simulink model "Inversor_full_bridge_ma"  (R2015a)
settings: Solver=ode23tb  StartTime=0.0  StopTime=0.2  MaxStep=0.5e-6  RelTol=1e-3
libraries: powerlib x11, simulink x1
settings Model: Creator=Leandro  LastModifiedBy=Iury
settings DataIOCC: SignalLoggingSaveFormat=ModelDataLogs
settings DebuggingCC: UnderspecifiedInitializationDetection=Classic  MergeDetectMultiDrivingBlocksExec=none  SolverPrmCheckMsg=warning  FcnCallInpInsideContextMsg=UseLocalSettings  StateNameClashWarn=warning
settings GRTTargetCC: CombineOutputUpdateFcns=off  GRTInterface=on

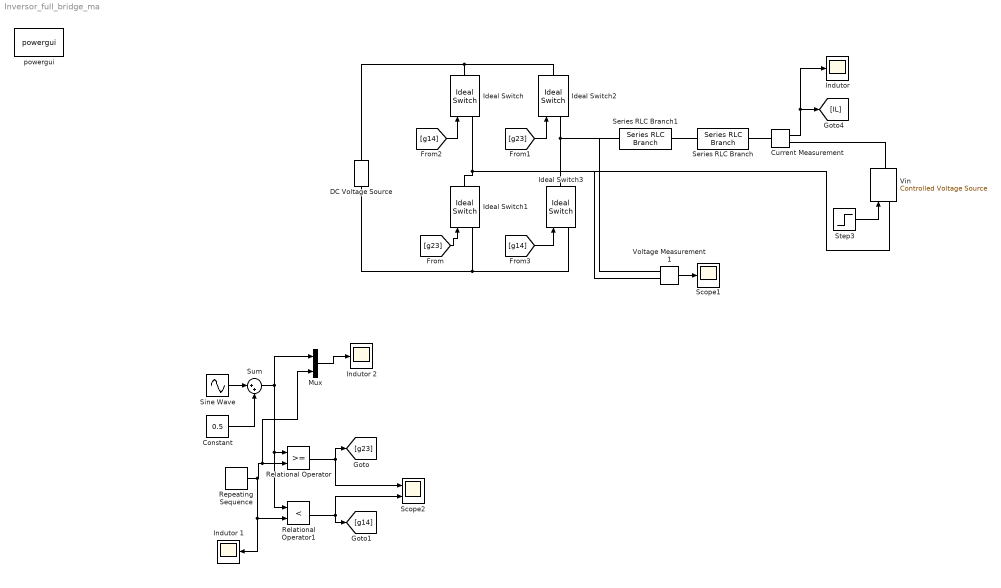
== system Inversor_full_bridge_ma ==
  Constant : Constant  Value=0.5
  Current Measurement : powerlib/Measurements/Current Measurement  PhasorSimulation=off  OutputType=Complex  PSBequivalent=0
  DC Voltage Source : powerlib/Electrical Sources/DC Voltage Source  Amplitude=200  Measurements=None
  Ideal Switch{,1..3} (4 alike) : powerlib/Power Electronics/Ideal Switch  Ron=1e-6  Lon=0  IC=0  Rs=1e5  Cs=inf  Measurements=off
  "Indutor " : Scope
      settings: TimeRange=0.05  YMin=0  YMax=20  SaveName=i
  Indutor 1 : Scope
      settings: TimeRange=0.05  YMin=0  YMax=20  SaveName=i1
  Indutor 2 : Scope
      settings: TimeRange=0.05  YMin=0  YMax=20  SaveName=i2
  Mux : Mux  Inputs=2
  Relational Operator : RelationalOperator  OutDataTypeStr=boolean
  Relational Operator1 : RelationalOperator  Operator=<  OutDataTypeStr=boolean
  Repeating Sequence : simulink/Sources/Repeating Sequence  rep_seq_t=[0 1/20000 1/10000]  rep_seq_y=[0 1 0]
  Scope1 : Scope
  Scope2 : Scope  NumInputPorts=2
      settings: TimeRange=0.05  YMin=0~0  YMax=1~1  SaveName=ScopeData2
  Series RLC Branch : powerlib/Elements/Series RLC Branch  LConnTagsString=__new0  RConnTagsString=__new0  BranchType=L  Resistance=0  Inductance=2e-3  SetiL0=off  InitialCurrent=0  Capacitance=1.0  Setx0=off  InitialVoltage=0  Measurements=None
  Series RLC Branch1 : powerlib/Elements/Series RLC Branch  LConnTagsString=__new0  RConnTagsString=__new0  BranchType=R  Resistance=0.1  Inductance=2e-3  SetiL0=off  InitialCurrent=0  Capacitance=1.0  Setx0=off  InitialVoltage=0  Measurements=None
  Sine Wave : Sin  Amplitude=0.3  Frequency=60*2*pi  SampleTime=0
  Step3 : Step  Time=0  After=0  SampleTime=0
  Sum : Sum  Inputs=|++
  Vin : powerlib/Electrical Sources/Controlled Voltage Source  Initialize=on  Source_Type=AC  Amplitude=0  Phase=0  Frequency=0  Measurements=None
  Voltage Measurement1 : powerlib/Measurements/Voltage Measurement  PhasorSimulation=off  OutputType=Complex  PSBequivalent=0
  powergui : powerlib/powergui  Priority=1  SimulationMode=Continuous  SolverType=Tustin  SampleTime=50e-6  frequency=60  SPID=on  DisableSnubberDevices=off  DisableRonSwitches=off  DisableVfSwitches=off  SwTol=0  DisplayEquations=off  Interpol=off  methode=off  Ts=0  FunctionMessages=off  echomessages=off  HookPort=off  EnableUseOfTLC=off  x0status=blocks  frequencyindice=0  Pbase=100e6  ErrMax=1e-4  Iterations=50  UnitsV=kV  UnitsW=MW  buscounter=0  RestoreLinks=warning  ResistiveCurrentMeasurement=off  Frange=[0:2:500]  Ylog=off  Xlog=on  ShowGrid=off  save=off  variable=ZData  structure=0  ZoomFFT=off  StartTime=0.0  cycles=1  DisplayStyle=1  fundamental=60  FreqAxis=off  MaxFrequency=1000  frequencyindicesteady=1  RmsSteady=1  display=off
  wires:
  Repeating Sequence/1 -> Indutor 1/1, Relational Operator1/2, Mux/2, Relational Operator/2
  Relational Operator/1 -> [g23], Scope2/1
  Relational Operator1/1 -> [g14], Scope2/2
  [g23] -> Ideal Switch1/1
  [g23] -> Ideal Switch2/1
  [g14] -> Ideal Switch/1
  [g14] -> Ideal Switch3/1
  Current Measurement/1 -> "Indutor "/1, [IL]
  Sine Wave/1 -> Sum/1
  Constant/1 -> Sum/2
  Sum/1 -> Relational Operator1/1, Relational Operator/1, Mux/1
  Mux/1 -> Indutor 2/1
  Voltage Measurement1/1 -> Scope1/1
  Step3/1 -> Vin/1
  connections:
  Series RLC Branch/RConn1 -- Current Measurement/LConn1
  Ideal Switch3/RConn1 -- Voltage Measurement1/LConn1 -- Series RLC Branch1/RConn1 -- Ideal Switch2/LConn1
  Ideal Switch2/RConn1 -- DC Voltage Source/RConn1 -- Ideal Switch/RConn1
  Ideal Switch3/LConn1 -- DC Voltage Source/LConn1 -- Ideal Switch1/LConn1
  Ideal Switch1/RConn1 -- Voltage Measurement1/LConn2 -- Vin/LConn1 -- Ideal Switch/LConn1
  Series RLC Branch1/LConn1 -- Series RLC Branch/LConn1
  Current Measurement/RConn1 -- Vin/RConn1
